simulink model "power_3phsignaldq"  (Simulink 6.0)
settings: Solver=FixedStepDiscrete  SolverMode=SingleTasking  StartTime=0.0  StopTime=0.15  MaxStep=200e-6  RelTol=1e-3  AbsTol=1e-2
libraries: powerlib_extras x5
settings Model: Creator=sybille  LastModifiedBy=batserve  ExtModeTrigMode=oneshot  ExtModeArmWhenConnect=off  ExtModeAutoUpdateStatusClock=off
settings DataIOCC: Decimation=10  LimitDataPoints=off  SaveFinalState=on  SaveOutput=off  SignalLoggingName=sigsOut
settings OptimizationCC: BlockReduction=off  BooleanDataType=off
settings DebuggingCC: CheckExecutionContextPreStartOutputMsg=on  CheckExecutionContextRuntimeOutputMsg=on  SolverPrmCheckMsg=none  UnconnectedInputMsg=none  UnconnectedOutputMsg=none
settings HardwareCC: TargetUnknown=on
settings RTWCC: TemplateMakefile=grt_vc.tmf

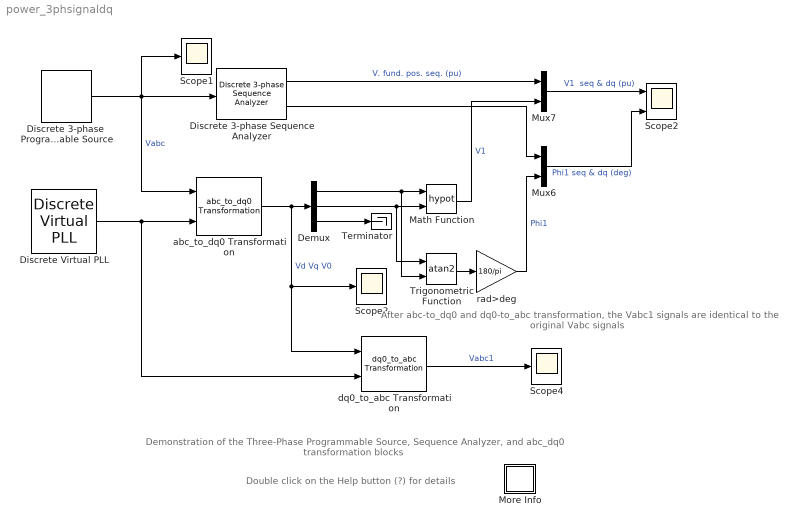
== system power_3phsignaldq ==
  note: Demonstration of the Three-Phase Programmable Source,  Sequence Analyzer,
      |  and  abc_dq0 transformation blocks
  note: After abc-to_dq0 and dq0-to_abc transformation,
      | the Vabc1 signals are identical to the original Vabc signals
  note: Double click on the Help button (?) for details
  Demux : Demux  Outputs=3
  Discrete 3-phase  Programmable Source : powerlib_extras/Discrete  Control Blocks/Discrete 3-phase  Programmable Source  Par_Vps="[1.0  15  60]"  VariationEntity=Amplitude  VariationType=Step  VariationStep=0.5  VariationRate=10  VariationMag=0.3  VariationFreq=2  Par_Timing_Variation=[0.05 1]  SinglePhase=on  Yampli=[1 0.2 1.2 1.0]  Xtime=[0 0.1 0.15 0.2]  HarmonicGeneration=on  Par_HarmoA=[1 0.3 -30 2]  Par_HarmoB=[1 0.0 0.0 1]  Par_Timing_Harmo="[0.1  1]"  Ts=50e-6
  Discrete Virtual PLL : powerlib_extras/Discrete  Control Blocks/Discrete Virtual PLL  Freq=60  Phase=0  Ts=50e-6
  Discrete 3-phase Sequence Analyzer : powerlib_extras/Discrete Measurements/Discrete 3-phase Sequence Analyzer  Freq=60  n=1  seq=Positive  Par_Init=[1 15]  Ts=50e-6
  Math Function : Math  Operator=hypot  SaturateOnIntegerOverflow=on
  More Info : Subsystem
      mask Display: disp('?')
  Mux6 : Mux  Inputs=2
  Mux7 : Mux  Inputs=2
  Scope1 : Scope
      settings: TickLabels=on  TimeRange=0.15  YMin=-2  YMax=2  DataFormat=Array  SampleInput=on
  Scope2 : Scope  NumInputPorts=2
      settings: TimeRange=0.15  YMin=1~0  YMax=2~30  DataFormat=Array  SampleInput=on
  Scope3 : Scope
      settings: TickLabels=on  TimeRange=0.16  YMin=-0.5  YMax=1.5  DataFormat=Array  SampleInput=on
  Scope4 : Scope
      settings: TickLabels=on  TimeRange=0.15  YMin=-1.5  YMax=1.5  DataFormat=Array  SampleInput=on
  Terminator : Terminator
  Trigonometric Function : Trigonometry  Operator=atan2
  abc_to_dq0 Transformation : powerlib_extras/Measurements/abc_to_dq0 Transformation
  dq0_to_abc Transformation : powerlib_extras/Measurements/dq0_to_abc Transformation
  rad>deg : Gain  Gain=180/pi  SaturateOnIntegerOverflow=on
  wires:
  Demux/2 -> Math Function/2, Trigonometric Function/1
  Demux/1 -> Math Function/1, Trigonometric Function/2
  Math Function/1 -> Mux7/2  "V1"
  Discrete 3-phase Sequence Analyzer/1 -> Mux7/1  "V. fund. pos. seq. (pu)"
  Discrete 3-phase Sequence Analyzer/2 -> Mux6/1
  abc_to_dq0 Transformation/1 -> Demux/1, Scope3/1, dq0_to_abc Transformation/1  "Vd Vq V0"
  Trigonometric Function/1 -> rad>deg/1
  rad>deg/1 -> Mux6/2  "Phi1"
  dq0_to_abc Transformation/1 -> Scope4/1  "Vabc1"
  Mux6/1 -> Scope2/2  "Phi1 seq & dq (deg)"
  Mux7/1 -> Scope2/1  "V1  seq & dq (pu)"
  Discrete 3-phase  Programmable Source/1 -> Scope1/1, Discrete 3-phase Sequence Analyzer/1, abc_to_dq0 Transformation/1  "Vabc"
  Discrete Virtual PLL/2 -> abc_to_dq0 Transformation/2, dq0_to_abc Transformation/2
  Demux/3 -> Terminator/1

== system power_3phsignaldq/More Info ==
  note: Choose Simulation/Start and observe the instantaneous signals Vabc on Scope,
      |  the signal magnitude (V1) and phase (Phi1)  returned by the Sequence Analyzer (Scope2)
      |  and the d, q and  0 components  displayed on Scope3.
      |
      | Note that the Sequence Analyzer using Fourier analysis is immune to harmonics and unbalance (yellow traces of Scope2).
      | However, its response to a step is a one-cycle ramp.
      |
      | The abc_dqo transformation is instantaneous.
      | However, the imbalance starting at 0.1 s produces a ripple at the V1 and Phi1 outputs (magenta traces of Scope2).
  note: Demonstration
  note: This demonstration ilustrates use of the Three-Phase Programmable Source,
      | abc_dq0, and Sequence Analyzer blocks
  note: System Description
  note: A Discrete 3-Phase ProgrammableSource block is used to generate a 1 pu, 15 degrees positive sequence voltage.
      | At t = 0.05 s the positive sequence voltage is increased to 1.5 pu.
      | At t = 0.1 s an unbalance is introduced by adding a 0.3 pu negative sequence component with a phase of -30 degrees.
      |
      | The magnitude and phase of the positive-sequence component is evaluated in two diiferent ways:
      | 1) Sequence calculation of phasors using Fourier analysis; and 2) abc to dq0 transformation.
      |
      | Math Function and Trigonometric Function blocks are used to evaluate the magnitude and phase
      | of the positive sequence  from the d and q components:
      |
      | V1 = sqrt(Vd^2 + Vq^2)  ,  Phi1 = atan(Vq/Vd))
  note: G. Sybille (Hydro-Quebec)
